simulink model "Debouncing"  (R2024b)
settings: Solver=VariableStepAuto  StartTime=0.0  StopTime=10.0  RelTol=1e-3
libraries: arduinolib x2
settings Model: Creator=Ahmad  LastModifiedBy=Ahmad

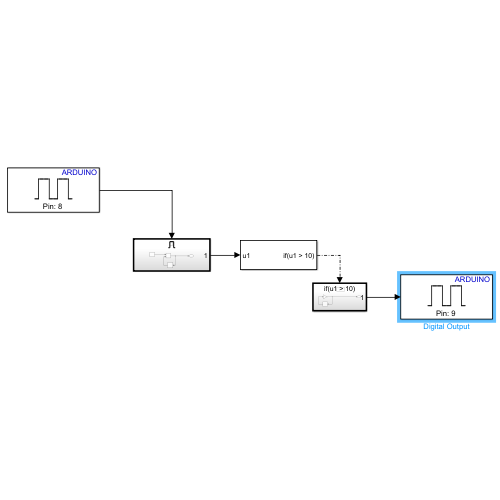
[thumbnail: Simulink's stored preview of the top-level diagram]
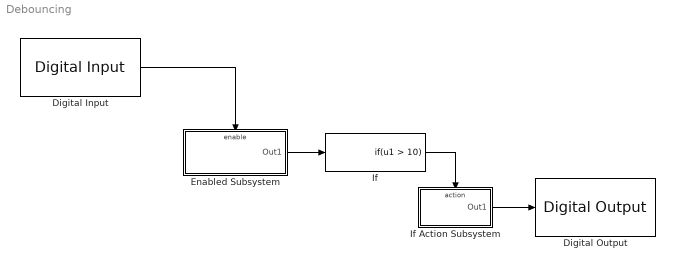
== system Debouncing ==
  Digital Input : arduinolib/Digital Input  pinNumber=8  mode=Default  Direction=input  SampleTime=0.1  blockPlatform=arduino
  Digital Output : arduinolib/Digital Output  pinNumber=9  Direction=output  blockPlatform=arduino
  Enabled Subsystem : Subsystem  TreatAsAtomicUnit=on
  If : If  IfExpression=u1 > 10  ShowElse=off
  If Action Subsystem : Subsystem  TreatAsAtomicUnit=on
  wires:
  Digital Input/1 -> Enabled Subsystem/Enable
  Enabled Subsystem/1(Out1) -> If/1
  If/1 -> If Action Subsystem/Action
  If Action Subsystem/1(Out1) -> Digital Output/1

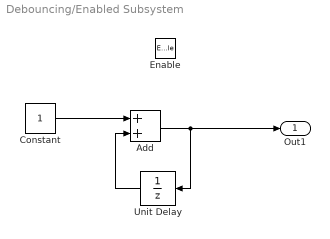
== system Debouncing/Enabled Subsystem ==
  Enable : EnablePort
  Add : Sum
  Constant : Constant
  Unit Delay : UnitDelay  SampleTime=-1  HasFrameUpgradeWarning=on
  Out1 : Outport
  wires:
  Constant/1 -> Add/1
  Add/1 -> Unit Delay/1, Out1/1
  Unit Delay/1 -> Add/2

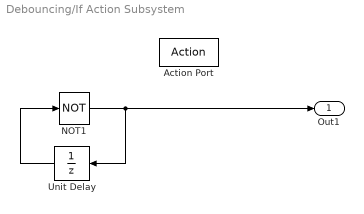
== system Debouncing/If Action Subsystem ==
  Action Port : ActionPort  ActionPortLabel=if(u1 > 10)
  NOT1 : Logic  Operator=NOT  IconShape=distinctive  AllPortsSameDT=off  OutDataTypeStr=boolean
  Unit Delay : UnitDelay  SampleTime=-1  HasFrameUpgradeWarning=on
  Out1 : Outport
  wires:
  NOT1/1 -> Unit Delay/1, Out1/1
  Unit Delay/1 -> NOT1/1
